simulink model "Control_try_2"  (R2021a)
settings: Solver=VariableStepAuto  StartTime=0.0  StopTime=inf  RelTol=1e-3
undefined symbols (not defined in the file or in its folder): DiscIntNeverNeededParam
libraries: mobileRoboticsLib x25
(part 2 of 2)

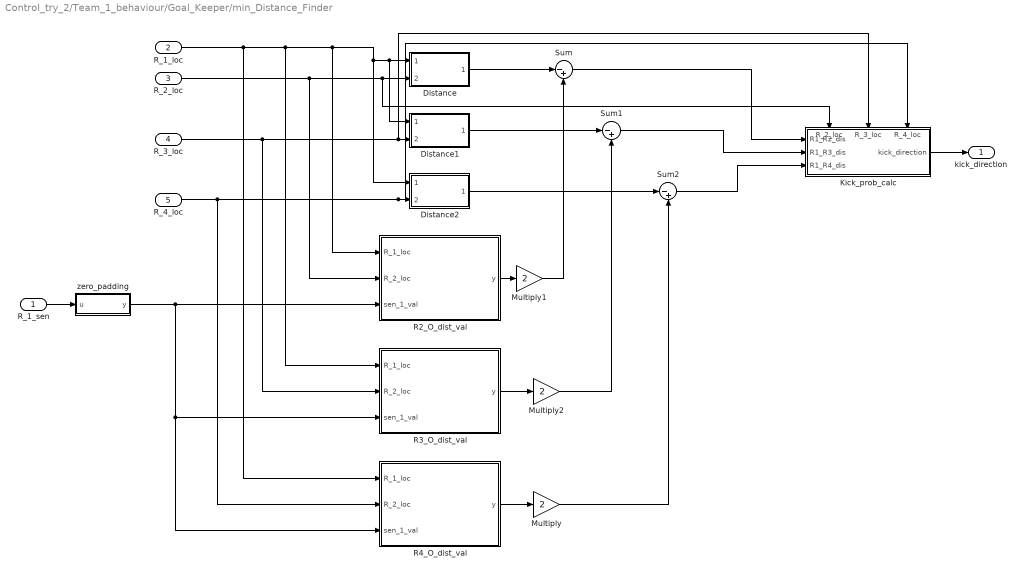
== system Control_try_2/Team_1_behaviour/Goal_Keeper/min_Distance_Finder ==
  R_1_sen : Inport
  R_1_loc : Inport  Port=2
  R_2_loc : Inport  Port=3
  R_3_loc : Inport  Port=4
  R_4_loc : Inport  Port=5
  Distance : Subsystem
  Distance1 : Subsystem
  Distance2 : Subsystem
  Kick_prob_calc : Stateflow chart  TreatAsAtomicUnit=on
      settings: PortSchema="{\"entries\":[{\"content\":{\"sides\":[{\"content\":{\"connectorIds\":[\"In4\",\"In5\",\"In6\"]},\"type\":\"ConnectorPlacement.EquallySpacedRectSide\",\"uuid\":\"64545375-395a-4478-8a53-b77c7ccd5016\"},{\"content\":{\"connectorIds\":[\"Out1\"],\"side\":\"RIGHT\"},\"type\":\"ConnectorPlacement.EquallySpacedRectSide\",\"uuid\":\"7cc0c28a-cc26-4f23-9952-6261e736221a\"},{\"content\":{\"connectorIds\":[\"In2\",\"In3\",\"In1\"],\"side\":\"TOP\"},\"type\":\"ConnectorPlacement.EquallySpacedRectSide\",\"uuid\":\"3f39c863-1804-4707-87c1-6f77798d874b\"},{\"content\":{\"connectorIds\":[],\"side\":\"BOTTOM\"},\"type\":\"ConnectorPlacement.EquallySpacedRectSide\",\"uuid\":\"dd00a5df-2ac1-49a5-bc9d-cbc3bc53305b\"}]},\"type\":\"ConnectorPlacement.EquallySpacedConnector\",\"uuid\":\"731ad359-9b43-4c19-839e-d6f1a372c8a6\"}],\"packageUris\":[\"http://schema.mathworks.com/mf0/Connector/R2020b\"],\"version\":\"1.0\"}"
  Multiply : Gain  Gain=2
  Multiply1 : Gain  Gain=2
  Multiply2 : Gain  Gain=2
  R2_O_dist_val : Subsystem
  R3_O_dist_val : Subsystem
  R4_O_dist_val : Subsystem
  Sum : Sum  Inputs=|-+
  Sum1 : Sum  Inputs=|-+
  Sum2 : Sum  Inputs=|-+
  zero_padding : MATLAB Function  TreatAsAtomicUnit=on
  kick_direction : Outport
  wires:
  R_2_loc/1 -> R2_O_dist_val/2(R_2_loc), Distance/2(R_2_loc), Kick_prob_calc/2(R_2_loc)
  R_1_loc/1 -> R4_O_dist_val/1(R_1_loc), R3_O_dist_val/1(R_1_loc), R2_O_dist_val/1(R_1_loc), Distance2/1(R_1_loc), Distance1/1(R_1_loc), Distance/1(R_1_loc)
  R_3_loc/1 -> R3_O_dist_val/2(R_2_loc), Distance1/2(R_3_loc), Kick_prob_calc/3(R_3_loc)
  R_4_loc/1 -> R4_O_dist_val/2(R_2_loc), Distance2/2(R_4_loc), Kick_prob_calc/1(R_4_loc)
  Kick_prob_calc/1(kick_direction) -> kick_direction/1
  R_1_sen/1 -> zero_padding/1(u)
  zero_padding/1(y) -> R3_O_dist_val/3(sen_1_val), R4_O_dist_val/3(sen_1_val), R2_O_dist_val/3(sen_1_val)
  R2_O_dist_val/1(y) -> Multiply1/1
  R3_O_dist_val/1(y) -> Multiply2/1
  R4_O_dist_val/1(y) -> Multiply/1
  Distance/1(R1_R2_dis) -> Sum/1
  Multiply1/1 -> Sum/2
  Distance1/1(R1_R3_dis) -> Sum1/1
  Distance2/1(R1_R4_dis) -> Sum2/1
  Multiply2/1 -> Sum1/2
  Multiply/1 -> Sum2/2
  Sum/1 -> Kick_prob_calc/4(R1_R2_dis)
  Sum1/1 -> Kick_prob_calc/5(R1_R3_dis)
  Sum2/1 -> Kick_prob_calc/6(R1_R4_dis)

== system Control_try_2/Team_1_behaviour/Goal_Keeper/kick_direction/Angle Finder1 ==
  In1 : Inport
  Abs : Abs
  Atan : Trigonometry  Operator=atan
  Demux : Demux  Outputs=2
  Divide : Product  Inputs=/*
  angle : Outport
  wires:
  Divide/1 -> Atan/1
  Demux/2 -> Divide/2
  Demux/1 -> Divide/1
  Atan/1 -> Abs/1
  Abs/1 -> angle/1
  In1/1 -> Demux/1

== system Control_try_2/Team_1_behaviour/Goal_Keeper/min_Distance_Finder/Distance ==
  R_1_loc : Inport
  R_2_loc : Inport  Port=2
  Demux : Demux  Outputs=3
  Demux1 : Demux  Outputs=3
  Square : Math  Operator=square  SaturateOnIntegerOverflow=on
  Square Root : Sqrt  SaturateOnIntegerOverflow=on
  Square1 : Math  Operator=square  SaturateOnIntegerOverflow=on
  Sum : Sum  Inputs=|+-
  Sum1 : Sum  Inputs=|+-
  Sum2 : Sum  Inputs=|++
  R1_R2_dis : Outport
  wires:
  Square1/1 -> Sum2/2
  Demux/2 -> Sum1/1
  Sum2/1 -> Square Root/1
  Square/1 -> Sum2/1
  Demux/1 -> Sum/1
  Sum1/1 -> Square1/1
  Demux1/2 -> Sum1/2
  Sum/1 -> Square/1
  Demux1/1 -> Sum/2
  R_1_loc/1 -> Demux/1
  R_2_loc/1 -> Demux1/1
  Square Root/1 -> R1_R2_dis/1

== system Control_try_2/Team_1_behaviour/Goal_Keeper/min_Distance_Finder/Distance1 ==
  R_1_loc : Inport
  R_3_loc : Inport  Port=2
  Demux : Demux  Outputs=3
  Demux1 : Demux  Outputs=3
  Square : Math  Operator=square  SaturateOnIntegerOverflow=on
  Square Root : Sqrt  SaturateOnIntegerOverflow=on
  Square1 : Math  Operator=square  SaturateOnIntegerOverflow=on
  Sum : Sum  Inputs=|+-
  Sum1 : Sum  Inputs=|+-
  Sum2 : Sum  Inputs=|++
  R1_R3_dis : Outport
  wires:
  Square1/1 -> Sum2/2
  Demux/2 -> Sum1/1
  Sum2/1 -> Square Root/1
  Square/1 -> Sum2/1
  Demux/1 -> Sum/1
  Sum1/1 -> Square1/1
  Demux1/2 -> Sum1/2
  Sum/1 -> Square/1
  Demux1/1 -> Sum/2
  R_1_loc/1 -> Demux/1
  R_3_loc/1 -> Demux1/1
  Square Root/1 -> R1_R3_dis/1

== system Control_try_2/Team_1_behaviour/Goal_Keeper/min_Distance_Finder/Distance2 ==
  R_1_loc : Inport
  R_4_loc : Inport  Port=2
  Demux : Demux  Outputs=3
  Demux1 : Demux  Outputs=3
  Square : Math  Operator=square  SaturateOnIntegerOverflow=on
  Square Root : Sqrt  SaturateOnIntegerOverflow=on
  Square1 : Math  Operator=square  SaturateOnIntegerOverflow=on
  Sum : Sum  Inputs=|+-
  Sum1 : Sum  Inputs=|+-
  Sum2 : Sum  Inputs=|++
  R1_R4_dis : Outport
  wires:
  Square1/1 -> Sum2/2
  Demux/2 -> Sum1/1
  Sum2/1 -> Square Root/1
  Square/1 -> Sum2/1
  Demux/1 -> Sum/1
  Sum1/1 -> Square1/1
  Demux1/2 -> Sum1/2
  Sum/1 -> Square/1
  Demux1/1 -> Sum/2
  R_1_loc/1 -> Demux/1
  R_4_loc/1 -> Demux1/1
  Square Root/1 -> R1_R4_dis/1

== system Control_try_2/Team_1_behaviour/Goal_Keeper/min_Distance_Finder/R2_O_dist_val ==
  R_1_loc : Inport
  R_2_loc : Inport  Port=2
  sen_1_val : Inport  Port=3
  Chart : Stateflow chart  TreatAsAtomicUnit=on
  y : Outport
  wires:
  sen_1_val/1 -> Chart/2(sen_1_val)
  R_1_loc/1 -> Chart/1(R_1_loc)
  R_2_loc/1 -> Chart/3(R_2_loc)
  Chart/1(dist) -> y/1

== system Control_try_2/Team_1_behaviour/Goal_Keeper/min_Distance_Finder/R3_O_dist_val ==
  R_1_loc : Inport
  R_2_loc : Inport  Port=2
  sen_1_val : Inport  Port=3
  Chart : Stateflow chart  TreatAsAtomicUnit=on
  y : Outport
  wires:
  Chart/1(dist) -> y/1
  R_2_loc/1 -> Chart/3(R_2_loc)
  R_1_loc/1 -> Chart/1(R_1_loc)
  sen_1_val/1 -> Chart/2(sen_1_val)

== system Control_try_2/Team_1_behaviour/Goal_Keeper/min_Distance_Finder/R4_O_dist_val ==
  R_1_loc : Inport
  R_2_loc : Inport  Port=2
  sen_1_val : Inport  Port=3
  Chart : Stateflow chart  TreatAsAtomicUnit=on
  y : Outport
  wires:
  sen_1_val/1 -> Chart/2(sen_1_val)
  R_1_loc/1 -> Chart/1(R_1_loc)
  R_2_loc/1 -> Chart/3(R_2_loc)
  Chart/1(dist) -> y/1

== stateflow chart Control_try_2/Referee/GOAL ==
  state Start
    en:
    right_team_goal = 0;
    left_team_goal = 0;
  state Goal_left
    en:
    right_team_goal = right_team_goal +1 ;
  state in_field
    en:
  state Goal_right
    en:
    left_team_goal = left_team_goal + 1;
  (default) -> Start
  Start -> in_field : [X > 1 && X<10 && Y > 1  && Y < 7]
  in_field -> Goal_left [order 2] : [fix(X) == 1 && Y > 2.7  && Y < 5.3 && Z < 1.2]
  Goal_right -> in_field : [X > 1 && X<10 && Y > 1  && Y < 7]
  in_field -> Goal_right [order 1] : [fix(X) == 10 && Y > 2.7  && Y < 5.3 && Z <1.2]
  Goal_left -> in_field : [X > 1 && X<10 && Y > 1  && Y < 7]
  data: X input; Y input; Z input; left_team_goal output; right_team_goal output

== stateflow chart Control_try_2/Referee/Throwin ==
  data: X input; Y input

== stateflow chart Control_try_2/Referee/Corner ==

== stateflow chart Control_try_2/Referee/Penelty ==

== matlab function Control_try_2/Enviornment/MATLAB Function ==

function plotEnvironment

coder.extrinsic('evalin');
persistent hasPlotted
if isempty(hasPlotted)
    evalin('base','environment_Plot');
    hasPlotted = true;
end

== stateflow chart Control_try_2/Enviornment/Ball_Dynamics/Chart ==
  state on_ground
    du:
    if(abs(F)>2.6)
    a = (abs(F)-2.6) * (F/abs(F)) / 0.43
    else
    a = 0
    end
  state off_ground
    du:
    a = F/0.43
  (default) -> on_ground
  off_ground -> on_ground : [Y ==0]
  on_ground -> off_ground : [Y > 0]
  data: Y input; F input; a output

== stateflow chart Control_try_2/Enviornment/Ball_Dynamics/Chart1 ==
  state calculations_neg
    du:
    vs = (abs(v))*(abs(v))*(-1)
  state calculations_pos
    du:
    vs = v*v
  (default) -> calculations_neg
  calculations_pos -> calculations_neg : [v<0]
  calculations_neg -> calculations_pos : [v>0]
  data: vs output; v input

== stateflow chart Control_try_2/Enviornment/Ball_Dynamics/Chart2 ==
  state on_ground
    du:
    if(abs(F)>2.6)
    a = (abs(F) - 2.6) * (F/abs(F)) / 0.43
    else
    a = 0
    end
  state off_ground
    du:
    a = F/0.43
  (default) -> on_ground
  off_ground -> on_ground : [Y ==0]
  on_ground -> off_ground : [Y > 0]
  data: Y input; F input; a output

== stateflow chart Control_try_2/Enviornment/Ball_Dynamics/Chart3 ==
  state calculations_neg
    du:
    vs = (abs(v))*(abs(v))*(-1)
  state calculations_pos
    du:
    vs = v*v
  (default) -> calculations_neg
  calculations_pos -> calculations_neg : [v<0]
  calculations_neg -> calculations_pos : [v>=0]
  data: vs output; v input

== stateflow chart Control_try_2/Enviornment/Ball_Dynamics/Chart4 ==
  state in_motion
    du:
    if (v > 0)
    a = -(0.32*0.98)
    else if(v<0)
    a = (0.32*0.98)
    end
    end
  state stationary
    du:
    a = 0;
  (default) -> in_motion
  in_motion -> stationary : [abs(v) < 0.03 | Y>0]
  stationary -> in_motion : [abs(v)>0.03]
  data: Y input; a output; v input

== stateflow chart Control_try_2/Team_1_behaviour/Goal_Keeper/control ==
  state Ball_Following
    du:
    kick = 0;
    if (R1_loc_Y>2.7 && R1_loc_Y<5.3)
    if(Ball_loc_Y > R1_loc_Y)
    R1_vel_Y = 0.04;
    else if (Ball_loc_Y < R1_loc_Y)
    R1_vel_Y = -0.04;
    end
    end
    else if ( R1_loc_Y > 5.3)
    R1_vel_Y = -0.04;
    else if ( R1_loc_Y < 2.7)
    R1_vel_Y = -0.04;
    end
    end
    end
  state Ball_Held
    du:
    kick = 1;
  (default) -> Ball_Following
  Ball_Following -> Ball_Held : [GB_dist < 0.15]
  Ball_Held -> Ball_Following : [GB_dist > 0.15]
  data: kick output; R1_loc_X input; Ball_loc_X input; GB_dist input; R1_loc_Y input; Ball_loc_Y input; R1_vel_Y output

== stateflow chart Control_try_2/Enviornment/Ball_Dynamics/Chart6 ==
  state in_motion
    du:
    if (v > 0)
    a = -(0.32*0.98)
    else if(v<0)
    a = (0.32*0.98)
    end
    end
  state stationary
    du:
    a = 0;
  (default) -> in_motion
  in_motion -> stationary : [abs(v) < 0.01 | Y>0]
  stationary -> in_motion : [abs(v)>0.02]
  data: Y input; a output; v input

== stateflow chart Control_try_2/Team_1_behaviour/Goal_Keeper/min_Distance_Finder/Kick_prob_calc ==
  state bot_2
    du:
    kick_direction = R_2_loc
  state bot_3
    du:
    kick_direction = R_3_loc
  state bot_4
    du:
    kick_direction = R_4_loc
  (default) -> bot_2
  bot_2 -> bot_3 [order 1] : [R1_R3_dis < R1_R2_dis && R1_R3_dis < R1_R4_dis]
  bot_3 -> bot_2 [order 1] : [R1_R2_dis < R1_R3_dis && R1_R2_dis < R1_R4_dis]
  bot_4 -> bot_2 [order 2] : [R1_R2_dis < R1_R3_dis && R1_R2_dis < R1_R4_dis]
  bot_2 -> bot_4 [order 2] : [R1_R4_dis < R1_R3_dis && R1_R4_dis < R1_R2_dis]
  bot_3 -> bot_4 [order 2] : [R1_R4_dis < R1_R3_dis && R1_R4_dis < R1_R2_dis]
  bot_4 -> bot_3 [order 1] : [R1_R3_dis < R1_R2_dis && R1_R3_dis < R1_R4_dis]
  data: R_4_loc input; R_2_loc input; R_3_loc input; R1_R2_dis input; R1_R3_dis input; R1_R4_dis input; kick_direction output

== stateflow chart Control_try_2/Team_1_behaviour/Goal_Keeper/min_Distance_Finder/R3_O_dist_val/Chart ==
  state calculate
    en:
    dist = 0;
    pos_x = 0;
    pos_y =0;
    dist_x =0;
    dist_y = 0;
    i=0;
    du:
    dist = 0;
    for i=1:7
    if (sen_1_val(i,3) > 4)
    pos_x = R_1_loc(1) + sen_1_val(i,1);
    pos_y = R_1_loc(2) + sen_1_val(i,2);
    dist_x = R_2_loc(1) - pos_x;
    dist_y = R_2_loc(2) - pos_y;
    dist = dist + sqrt((dist_x*dist_x) + (dist_y*dist_y));
    end
    end
  (default) -> calculate
  data: R_1_loc input; sen_1_val input; dist output; R_2_loc input; dist_y local; i local; pos_x local; pos_y local; dist_x local

== stateflow chart Control_try_2/Team_1_behaviour/Goal_Keeper/min_Distance_Finder/R2_O_dist_val/Chart ==
  state calculate
    en:
    dist = 0;
    pos_x = 0;
    pos_y =0;
    dist_x =0;
    dist_y = 0;
    i=0;
    du:
    dist = 0;
    for i=1:7
    if (sen_1_val(i,3) > 4)
    pos_x = R_1_loc(1) + sen_1_val(i,1);
    pos_y = R_1_loc(2) + sen_1_val(i,2);
    dist_x = R_2_loc(1) - pos_x;
    dist_y = R_2_loc(2) - pos_y;
    dist = dist + sqrt((dist_x*dist_x) + (dist_y*dist_y));
    end
    end
  (default) -> calculate
  data: R_1_loc input; sen_1_val input; dist output; R_2_loc input; dist_y local; i local; pos_x local; pos_y local; dist_x local

== stateflow chart Control_try_2/Team_1_behaviour/Goal_Keeper/min_Distance_Finder/R4_O_dist_val/Chart ==
  state calculate
    en:
    dist = 0;
    pos_x = 0;
    pos_y =0;
    dist_x =0;
    dist_y = 0;
    i=0;
    du:
    dist = 0;
    for i=1:7
    if (sen_1_val(i,3) > 4)
    pos_x = R_1_loc(1) + sen_1_val(i,1);
    pos_y = R_1_loc(2) + sen_1_val(i,2);
    dist_x = R_2_loc(1) - pos_x;
    dist_y = R_2_loc(2) - pos_y;
    dist = dist + sqrt((dist_x*dist_x) + (dist_y*dist_y));
    end
    end
  (default) -> calculate
  data: R_1_loc input; sen_1_val input; dist output; R_2_loc input; dist_y local; i local; pos_x local; pos_y local; dist_x local

== stateflow chart Control_try_2/Team_1_behaviour/Goal_Keeper/kick_direction/Chart1 ==
  state x_pos
    du:
    Vx = 1
  state x_neg
    du:
    Vx = -1
  (default) -> x_pos
  x_pos -> x_neg : [x > 0]
  x_neg -> x_pos : [x<1]
  data: Vx output; x input

== stateflow chart Control_try_2/Team_1_behaviour/Goal_Keeper/kick_direction/Chart2 ==
  state y_pos
    du:
    Vy = 1
  state y_neg
    du:
    Vy = -1
  (default) -> y_pos
  y_pos -> y_neg : [y > 0]
  y_neg -> y_pos : [y<1]
  data: y input; Vy output

== matlab function Control_try_2/Team_1_behaviour/Goal_Keeper/min_Distance_Finder/zero_padding ==
  data: u input; y output
function y = pad(u)
% Zero-pads object detections to work with arrays of buses

y = zeros(7,3);
numElems = min(size(u,1),7);
for idx = 1:numElems
   y(idx,1:3) = u(idx,1:3); 
end
end

== stateflow chart Control_try_2/Team 1 Behaviour/Chart4 ==
  state second_coordinate
    du:
    actual_angle = -pi +angle + angle_bot;
  state first_coordinate
    du:
    actual_angle = angle_bot - angle;
  state ffourth_coordinate
    du:
    actual_angle = -(2*pi) + angle + angle_bot
  state Third_coordinate
    du:
    actual_angle =-(pi) - angle + angle_bot;
  (default) -> first_coordinate
  first_coordinate -> second_coordinate [order 1] : [ Rx>Bx && Ry<By ]
  second_coordinate -> first_coordinate [order 1] : [ Rx<Bx && Ry<By]
  ffourth_coordinate -> second_coordinate [order 1] : [ Rx>Bx && Ry<By ]
  first_coordinate -> Third_coordinate [order 3] : [ Rx>Bx && Ry>By]
  second_coordinate -> Third_coordinate [order 3] : [ Rx>Bx && Ry>By ]
  Third_coordinate -> second_coordinate [order 1] : [ Rx>Bx && Ry<By ]
  second_coordinate -> ffourth_coordinate [order 2] : [ Rx<Bx && Ry>By ]
  Third_coordinate -> first_coordinate [order 2] : [ Rx<Bx && Ry<By ]
  ffourth_coordinate -> first_coordinate [order 2] : [ Rx<Bx && Ry<By ]
  first_coordinate -> ffourth_coordinate [order 2] : [ Rx<Bx && Ry>By ]
  Third_coordinate -> ffourth_coordinate [order 3] : [ Rx<Bx && Ry>By ]
  ffourth_coordinate -> Third_coordinate [order 3] : [ Rx>Bx && Ry>By]
  data: Bx input; By input; Rx input; Ry input; angle input; actual_angle output; angle_bot input

== stateflow chart Control_try_2/Team 1 Behaviour/Chart5 ==
  state stop
    du:
    w = 0;
    v=0.25 * velocity;
  state RCW
    du:
    w = -1*1;
    v=0;
  state RCCW
    du:
    w =1*1;
    v=0;
  (default) -> stop
  stop -> RCCW [order 2] : [after(1,sec) && DT > 0]
  stop -> RCW [order 1] : [after(1,sec) && DT < 0]
  RCW -> stop [order 1] : [DT<= 0.1 && DT>= -0.1]
  RCCW -> stop [order 1] : [DT<= 0.1 && DT>= -0.1]
  RCCW -> RCW [order 2] : [DT>0]
  RCW -> RCCW [order 2] : [DT<0]
  data: velocity input; v output; DT input; w output

== stateflow chart Control_try_2/Team 1 Behaviour/Velocity_Decider2 ==
  state Robot_Far
    du:
    velocity = 1;
    kick = 0;
  state Robot_Close
    du:
    velocity = 0;
    kick = 1;
  (default) -> Robot_Far
  Robot_Far -> Robot_Close : [DBR <= 0.25]
  Robot_Close -> Robot_Far : [DBR > 0.25]
  data: kick output; DBR input; velocity output

== stateflow chart Control_try_2/Team 1 Behaviour/kick_direction2/Chart1 ==
  state x_pos
    du:
    Vx = 1
  state x_neg
    du:
    Vx = -1
  (default) -> x_pos
  x_pos -> x_neg : [x > 0]
  x_neg -> x_pos : [x<1]
  data: Vx output; x input

== stateflow chart Control_try_2/Team 1 Behaviour/kick_direction2/Chart2 ==
  state y_pos
    du:
    Vy = 1
  state y_neg
    du:
    Vy = -1
  (default) -> y_pos
  y_pos -> y_neg : [y > 0]
  y_neg -> y_pos : [y<1]
  data: y input; Vy output

== stateflow chart Control_try_2/Team 1 Behaviour/kick_direction/Chart1 ==
  state x_pos
    du:
    Vx = 1
  state x_neg
    du:
    Vx = -1
  (default) -> x_pos
  x_pos -> x_neg : [x > 0]
  x_neg -> x_pos : [x<1]
  data: Vx output; x input

== stateflow chart Control_try_2/Team 1 Behaviour/Chart6 ==
  state second_coordinate
    du:
    actual_angle = -pi +angle + angle_bot;
  state first_coordinate
    du:
    actual_angle = angle_bot - angle;
  state ffourth_coordinate
    du:
    actual_angle = -(2*pi) + angle + angle_bot
  state Third_coordinate
    du:
    actual_angle =-(pi) - angle + angle_bot;
  (default) -> first_coordinate
  first_coordinate -> second_coordinate [order 1] : [ Rx>Bx && Ry<By ]
  second_coordinate -> first_coordinate [order 1] : [ Rx<Bx && Ry<By]
  ffourth_coordinate -> second_coordinate [order 1] : [ Rx>Bx && Ry<By ]
  first_coordinate -> Third_coordinate [order 3] : [ Rx>Bx && Ry>By]
  second_coordinate -> Third_coordinate [order 3] : [ Rx>Bx && Ry>By ]
  Third_coordinate -> second_coordinate [order 1] : [ Rx>Bx && Ry<By ]
  second_coordinate -> ffourth_coordinate [order 2] : [ Rx<Bx && Ry>By ]
  Third_coordinate -> first_coordinate [order 2] : [ Rx<Bx && Ry<By ]
  ffourth_coordinate -> first_coordinate [order 2] : [ Rx<Bx && Ry<By ]
  first_coordinate -> ffourth_coordinate [order 2] : [ Rx<Bx && Ry>By ]
  Third_coordinate -> ffourth_coordinate [order 3] : [ Rx<Bx && Ry>By ]
  ffourth_coordinate -> Third_coordinate [order 3] : [ Rx>Bx && Ry>By]
  data: Bx input; By input; Rx input; Ry input; angle input; actual_angle output; angle_bot input

== stateflow chart Control_try_2/Team 1 Behaviour/Chart7 ==
  state stop
    du:
    w = 0;
    v=0.25 * velocity;
  state RCW
    du:
    w = -1*1;
    v=0;
  state RCCW
    du:
    w =1*1;
    v=0;
  (default) -> stop
  stop -> RCCW [order 2] : [after(1,sec) && DT > 0]
  stop -> RCW [order 1] : [after(1,sec) && DT < 0]
  RCW -> stop [order 1] : [DT<= 0.1 && DT>= -0.1]
  RCCW -> stop [order 1] : [DT<= 0.1 && DT>= -0.1]
  RCCW -> RCW [order 2] : [DT>0]
  RCW -> RCCW [order 2] : [DT<0]
  data: velocity input; v output; DT input; w output

== stateflow chart Control_try_2/Team 1 Behaviour/Velocity_Decider3 ==
  state Robot_Far
    du:
    velocity = 1;
    kick = 0;
  state Robot_Close
    du:
    velocity = 0;
    kick = 1;
  (default) -> Robot_Far
  Robot_Far -> Robot_Close : [DBR <= 0.25]
  Robot_Close -> Robot_Far : [DBR > 0.25]
  data: kick output; DBR input; velocity output

== stateflow chart Control_try_2/Team 1 Behaviour/kick_direction3/Chart1 ==
  state x_pos
    du:
    Vx = 1
  state x_neg
    du:
    Vx = -1
  (default) -> x_pos
  x_pos -> x_neg : [x > 0]
  x_neg -> x_pos : [x<1]
  data: Vx output; x input

== stateflow chart Control_try_2/Team 1 Behaviour/kick_direction3/Chart2 ==
  state y_pos
    du:
    Vy = 1
  state y_neg
    du:
    Vy = -1
  (default) -> y_pos
  y_pos -> y_neg : [y > 0]
  y_neg -> y_pos : [y<1]
  data: y input; Vy output

== matlab function Control_try_2/Enviornment/Subsystem/MATLAB Function ==
  data: x output; x1 input; y output; y1 input; z1 input; k1 input; x2 input; y2 input; z2 input; k2 input; x3 input; y3 input; z3 input; k3 input; z output; k output; n output
function [x,y,z,k,n] = fcn(x1,y1,z1,k1,x2,y2,z2,k2,x3,y3,z3,k3)
    
    xs = [x1,x2,x3] ;
    ys = [y1,y2,y3] ;
    zs = [z1,z2,z3] ;
    ks = [k1,k2,k3] ;
   
    for i = 1:3
        if k(i) == 1
            x = xs(i) ;
            y = ys(i) ;
            z = zs(i) ;
            k = ks(i) ;
            n = i ;
        else
            x = 0 ;
            y = 0 ;
            z = 0 ;
            k = 0 ;
            n = 0 ;
        end
        if n > 0
            a = 0 ;
            while a < 1000
                a=a+1;
            end
        end
    end
   
end

== stateflow chart Control_try_2/Team 1 Behaviour/kick_direction/Chart2 ==
  state y_pos
    du:
    Vy = 1
  state y_neg
    du:
    Vy = -1
  (default) -> y_pos
  y_pos -> y_neg : [y > 0]
  y_neg -> y_pos : [y<1]
  data: y input; Vy output

== stateflow chart Control_try_2/Team 1 Behaviour/Velocity_Decider ==
  state Robot_Far
    du:
    velocity = 1;
    kick = 0;
  state Robot_Close
    du:
    velocity = 0;
    kick = 1;
  (default) -> Robot_Far
  Robot_Far -> Robot_Close : [DBR <= 0.25]
  Robot_Close -> Robot_Far : [DBR > 0.25]
  data: kick output; DBR input; velocity output

== stateflow chart Control_try_2/Team 1 Behaviour/Chart ==
  state second_coordinate
    du:
    actual_angle = -pi +angle + angle_bot;
  state first_coordinate
    du:
    actual_angle = angle_bot - angle;
  state ffourth_coordinate
    du:
    actual_angle = -(2*pi) + angle + angle_bot
  state Third_coordinate
    du:
    actual_angle =-(pi) - angle + angle_bot;
  (default) -> first_coordinate
  first_coordinate -> second_coordinate [order 1] : [ Rx>Bx && Ry<By ]
  second_coordinate -> first_coordinate [order 1] : [ Rx<Bx && Ry<By]
  ffourth_coordinate -> second_coordinate [order 1] : [ Rx>Bx && Ry<By ]
  first_coordinate -> Third_coordinate [order 3] : [ Rx>Bx && Ry>By]
  second_coordinate -> Third_coordinate [order 3] : [ Rx>Bx && Ry>By ]
  Third_coordinate -> second_coordinate [order 1] : [ Rx>Bx && Ry<By ]
  second_coordinate -> ffourth_coordinate [order 2] : [ Rx<Bx && Ry>By ]
  Third_coordinate -> first_coordinate [order 2] : [ Rx<Bx && Ry<By ]
  ffourth_coordinate -> first_coordinate [order 2] : [ Rx<Bx && Ry<By ]
  first_coordinate -> ffourth_coordinate [order 2] : [ Rx<Bx && Ry>By ]
  Third_coordinate -> ffourth_coordinate [order 3] : [ Rx<Bx && Ry>By ]
  ffourth_coordinate -> Third_coordinate [order 3] : [ Rx>Bx && Ry>By]
  data: Bx input; By input; Rx input; Ry input; angle input; actual_angle output; angle_bot input

== stateflow chart Control_try_2/Team 1 Behaviour/Chart3 ==
  state stop
    du:
    w = 0;
    v=0.25 * velocity;
  state RCW
    du:
    w = -1*1;
    v=0;
  state RCCW
    du:
    w =1*1;
    v=0;
  (default) -> stop
  stop -> RCCW [order 2] : [after(1,sec) && DT > 0]
  stop -> RCW [order 1] : [after(1,sec) && DT < 0]
  RCW -> stop [order 1] : [DT<= 0.1 && DT>= -0.1]
  RCCW -> stop [order 1] : [DT<= 0.1 && DT>= -0.1]
  RCCW -> RCW [order 2] : [DT>0]
  RCW -> RCCW [order 2] : [DT<0]
  data: velocity input; v output; DT input; w output
